simulink model "dsincos"  (R2017a)
settings: Solver=VariableStepAuto  StartTime=0.0  StopTime=10.0  RelTol=1e-3
libraries: autodiff x2, simulink x1
settings Model: Creator=eruffaldi  LastModifiedBy=eruffaldi

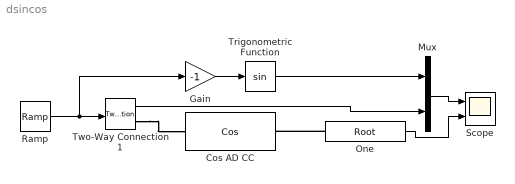
== system dsincos ==
  Cos AD CC : autodiff/Memberwise Scalar/Cos  SystemSampleTime=-1
      settings: SourceProductName=AutoDiff
  Gain : Gain  Gain=-1
  Mux : Mux  Inputs=2
  One : autodiff/Common/Root  SystemSampleTime=-1
      settings: SourceProductName=AutoDiff
  Ramp : simulink/Sources/Ramp  slope=1  start=0  X0=0
  Scope : Scope  NumInputPorts=2
  Trigonometric Function : Trigonometry
  Two-Way Connection1 : TwoWayConnection
  wires:
  Gain/1 -> Trigonometric Function/1
  Ramp/1 -> Gain/1, Two-Way Connection1/1
  Mux/1 -> Scope/1
  Trigonometric Function/1 -> Mux/1
  Two-Way Connection1/1 -> Mux/2
  One/1 -> Scope/2
  connections:
  Two-Way Connection1/RConn1 -- Cos AD CC/LConn1
  One/LConn1 -- Cos AD CC/RConn1
